simulink model "Distrubted_Settling_IO"  (R2021b)
settings: Solver=ode15s  StartTime=0.0  StopTime=600  FixedStep=0.01  RelTol=1e-5  AbsTol=1e-8
undefined symbols (not defined in the file or in its folder): Split_1_1, Split_2_1
settings Model: Creator=ielulf  LastModifiedBy=javanmcguckin
settings SolverCC: AutoScaleAbsTol=off  AlgebraicLoopSolver=TrustRegion
settings DataIOCC: InitialState=xFinal  SaveFormat=Array  SignalLoggingSaveFormat=ModelDataLogs  SaveOutput=off  ReturnWorkspaceOutputs=off  TimeSaveName=t  SignalLoggingName=sigsOut  OutputTimes=[0:(1/96):609]
settings OptimizationCC: BlockReduction=off  BooleanDataType=off  OptimizeBlockIOStorage=off  BufferReuse=off  GlobalBufferReuse=off  ExpressionFolding=off  ExpressionDepthLimit=2147483647  LocalBlockOutputs=off  InitFltsAndDblsToZero=on  LifeSpan=inf
settings DebuggingCC: SaveWithParameterizedLinksMsg=none  UnderspecifiedInitializationDetection=Classic  MergeDetectMultiDrivingBlocksExec=none  SignalResolutionControl=TryResolveAllWithWarning  InheritedTsInSrcMsg=none  MultiTaskDSMMsg=warning  MultiTaskCondExecSysMsg=none  FcnCallInpInsideContextMsg=warning  UnconnectedOutputMsg=none  StateNameClashWarn=warning  SFUnexpectedBacktrackingDiag=warning  SFNoUnconditionalDefaultTransitionDiag=warning  SFExecutionAtInitializationDiag=none  SFMachineParentedDataDiag=warning  ArithmeticOperatorsInVariantConditions=warning
settings HardwareCC: ProdBitPerPointer=32  ProdBitPerSizeT=32  ProdBitPerPtrDiffT=32  ProdLargestAtomicFloat=None  ProdIntDivRoundTo=Undefined  ProdEndianess=Unspecified  ProdWordSize=32  ProdHWDeviceType=32-bit Generic  TargetUnknown=on
settings ModelReferenceCC: PropagateSignalLabelsOutOfModel=off
settings SFSimCC: SimUseLocalCustomCode=off  CustomCodeUndefinedFunction=UseInterfaceOnly
settings RTWCC: TemplateMakefile=grt_unix.tmf  RTWUseLocalCustomCode=off
settings CodeAppCC: StateflowObjectComments=on
settings GRTTargetCC: TargetFcnLib=ansi_tfl_tmw.mat  TargetLangStandard=C89/C90 (ANSI)  CombineOutputUpdateFcns=off  GRTInterface=on
settings ConfigComp: CovMetricSettings=dw  CovSaveCumulativeToWorkspaceVar=on  CovSaveSingleToWorkspaceVar=on  CovExternalEMLEnable=off

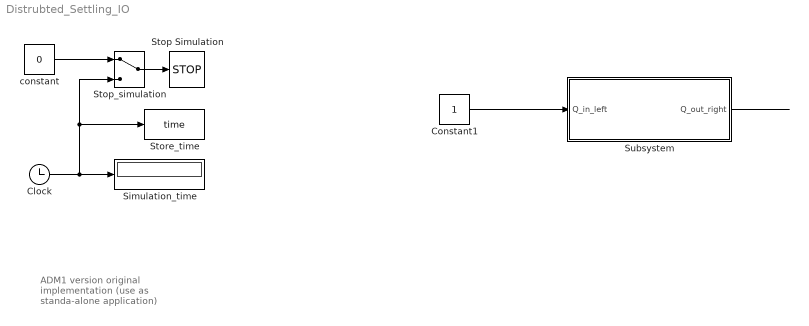
== system Distrubted_Settling_IO ==
  note: ADM1 version
      | original implementation
      | (use as standa-alone application)
  " constant" : Constant  Value=0
  Clock : Clock
  Constant1 : Constant
  Simulation_time : Display
  Stop Simulation : Stop
  Stop_simulation : ManualSwitch
  Store_time : ToWorkspace  VariableName=time
  Subsystem : Subsystem
  wires:
  Clock/1 -> Simulation_time/1, Stop_simulation/2, Store_time/1
  Stop_simulation/1 -> Stop Simulation/1
  " constant"/1 -> Stop_simulation/1
  Constant1/1 -> Subsystem/1(Q_in_left)
  Subsystem/1(Q_out_right) -> ?

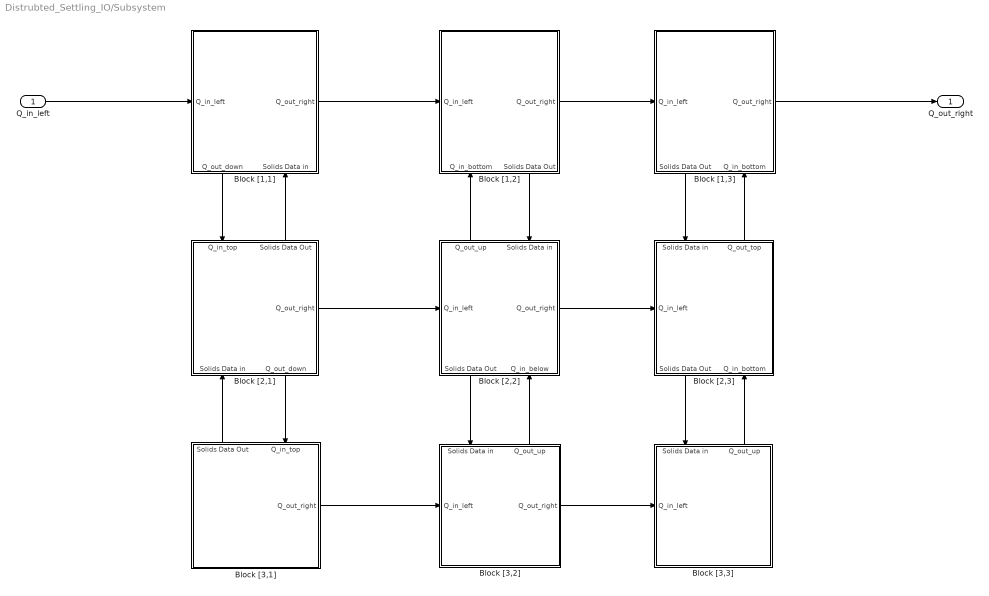
== system Distrubted_Settling_IO/Subsystem ==
  Q_in_left : Inport
  Block [1,1] : Subsystem
      settings: PortSchema="{\"entries\":[{\"content\":{\"sides\":[{\"content\":{\"connectorIds\":[\"In1\"]},\"type\":\"ConnectorPlacement.EquallySpacedRectSide\",\"uuid\":\"2b9ec2c5-2346-4716-8f77-26cfae708b75\"},{\"content\":{\"connectorIds\":[\"Out1\"],\"side\":\"RIGHT\"},\"type\":\"ConnectorPlacement.EquallySpacedRectSide\",\"uuid\":\"6f8825a3-51a4-4a9b-b2dd-ef4b1cf0d0ba\"},{\"content\":{\"connectorIds\":[],\"side\":\"TOP\"},\"type\":\"ConnectorPlacement.EquallySpacedRectSide\",\"uuid\":\"b45032d4-615e-469b-9b78-89fa084c4375\"},{\"content\":{\"connectorIds\":[\"Out2\",\"In2\"],\"side\":\"BOTTOM\"},\"type\":\"ConnectorPlacement.EquallySpacedRectSide\",\"uuid\":\"d5d8c6f1-1ff5-49da-af34-fac996f1665a\"}]},\"type\":\"ConnectorPlacement.EquallySpacedConnector\",\"uuid\":\"ae12b195-59d8-427e-9be1-69bc4b3728a5\"}],\"packageUris\":[\"http://schema.mathworks.com/mf0/Connector/R2020b\"],\"version\":\"1.0\"}"
  Block [1,2] : Subsystem
      settings: PortSchema="{\"entries\":[{\"content\":{\"sides\":[{\"content\":{\"connectorIds\":[\"In1\"]},\"type\":\"ConnectorPlacement.EquallySpacedRectSide\",\"uuid\":\"2b9ec2c5-2346-4716-8f77-26cfae708b75\"},{\"content\":{\"connectorIds\":[\"Out1\"],\"side\":\"RIGHT\"},\"type\":\"ConnectorPlacement.EquallySpacedRectSide\",\"uuid\":\"6f8825a3-51a4-4a9b-b2dd-ef4b1cf0d0ba\"},{\"content\":{\"connectorIds\":[],\"side\":\"TOP\"},\"type\":\"ConnectorPlacement.EquallySpacedRectSide\",\"uuid\":\"b45032d4-615e-469b-9b78-89fa084c4375\"},{\"content\":{\"connectorIds\":[\"In2\",\"Out2\"],\"side\":\"BOTTOM\"},\"type\":\"ConnectorPlacement.EquallySpacedRectSide\",\"uuid\":\"c255c3dc-4fb4-4a4d-908b-3c1bba827588\"}]},\"type\":\"ConnectorPlacement.EquallySpacedConnector\",\"uuid\":\"ae12b195-59d8-427e-9be1-69bc4b3728a5\"}],\"packageUris\":[\"http://schema.mathworks.com/mf0/Connector/R2020b\"],\"version\":\"1.0\"}"
  Block [1,3] : Subsystem
      settings: PortSchema="{\"entries\":[{\"content\":{\"sides\":[{\"content\":{\"connectorIds\":[\"In1\"]},\"type\":\"ConnectorPlacement.EquallySpacedRectSide\",\"uuid\":\"2b9ec2c5-2346-4716-8f77-26cfae708b75\"},{\"content\":{\"connectorIds\":[\"Out1\"],\"side\":\"RIGHT\"},\"type\":\"ConnectorPlacement.EquallySpacedRectSide\",\"uuid\":\"6f8825a3-51a4-4a9b-b2dd-ef4b1cf0d0ba\"},{\"content\":{\"connectorIds\":[],\"side\":\"TOP\"},\"type\":\"ConnectorPlacement.EquallySpacedRectSide\",\"uuid\":\"b45032d4-615e-469b-9b78-89fa084c4375\"},{\"content\":{\"connectorIds\":[\"Out2\",\"In2\"],\"side\":\"BOTTOM\"},\"type\":\"ConnectorPlacement.EquallySpacedRectSide\",\"uuid\":\"c6fd4661-f5fa-4e09-ac4d-c40a325ebb1e\"}]},\"type\":\"ConnectorPlacement.EquallySpacedConnector\",\"uuid\":\"ae12b195-59d8-427e-9be1-69bc4b3728a5\"}],\"packageUris\":[\"http://schema.mathworks.com/mf0/Connector/R2020b\"],\"version\":\"1.0\"}"
  Block [2,1] : Subsystem
      settings: PortSchema="{\"entries\":[{\"content\":{\"sides\":[{\"content\":{\"connectorIds\":[]},\"type\":\"ConnectorPlacement.EquallySpacedRectSide\",\"uuid\":\"3629ef0d-6d1b-4007-aa46-2d78e3d7de39\"},{\"content\":{\"connectorIds\":[\"Out1\"],\"side\":\"RIGHT\"},\"type\":\"ConnectorPlacement.EquallySpacedRectSide\",\"uuid\":\"902c1b28-6e40-40dc-9ba4-02f520de612f\"},{\"content\":{\"connectorIds\":[\"In1\",\"Out3\"],\"side\":\"TOP\"},\"type\":\"ConnectorPlacement.EquallySpacedRectSide\",\"uuid\":\"32048d77-21e8-4d7f-b37a-aa0fba1296d3\"},{\"content\":{\"connectorIds\":[\"In2\",\"Out2\"],\"side\":\"BOTTOM\"},\"type\":\"ConnectorPlacement.EquallySpacedRectSide\",\"uuid\":\"7ea0cf0e-949f-46a7-b1ef-2c29e41bdeea\"}]},\"type\":\"ConnectorPlacement.EquallySpacedConnector\",\"uuid\":\"783f8f0c-f046-4b3b-a07c-ac2bcfa72a90\"}],\"packageUris\":[\"http://schema.mathworks.com/mf0/Connector/R2020b\"],\"version\":\"1.0\"}"
  Block [2,2] : Subsystem
      settings: PortSchema="{\"entries\":[{\"content\":{\"sides\":[{\"content\":{\"connectorIds\":[\"In1\"]},\"type\":\"ConnectorPlacement.EquallySpacedRectSide\",\"uuid\":\"49108942-846e-4f10-a565-9a363346b2ee\"},{\"content\":{\"connectorIds\":[\"Out1\"],\"side\":\"RIGHT\"},\"type\":\"ConnectorPlacement.EquallySpacedRectSide\",\"uuid\":\"12efabec-6f68-4acd-88b6-a333148dee6c\"},{\"content\":{\"connectorIds\":[\"Out3\",\"In2\"],\"side\":\"TOP\"},\"type\":\"ConnectorPlacement.EquallySpacedRectSide\",\"uuid\":\"4d5dbabd-8754-411c-8b88-a1dca35fc46d\"},{\"content\":{\"connectorIds\":[\"Out2\",\"In3\"],\"side\":\"BOTTOM\"},\"type\":\"ConnectorPlacement.EquallySpacedRectSide\",\"uuid\":\"6311604b-5e77-49d3-b6da-7ee01c36d0f1\"}]},\"type\":\"ConnectorPlacement.EquallySpacedConnector\",\"uuid\":\"2bdac1b1-172b-46d0-a20b-b916e0c0b218\"}],\"packageUris\":[\"http://schema.mathworks.com/mf0/Connector/R2020b\"],\"version\":\"1.0\"}"
  Block [2,3] : Subsystem
      settings: PortSchema="{\"entries\":[{\"content\":{\"sides\":[{\"content\":{\"connectorIds\":[\"In1\"]},\"type\":\"ConnectorPlacement.EquallySpacedRectSide\",\"uuid\":\"482fbcbb-9155-4fc8-9601-0ed92cde34b4\"},{\"content\":{\"connectorIds\":[],\"side\":\"RIGHT\"},\"type\":\"ConnectorPlacement.EquallySpacedRectSide\",\"uuid\":\"966a36b1-158b-4266-8167-7a28a80d741e\"},{\"content\":{\"connectorIds\":[\"In2\",\"Out2\"],\"side\":\"TOP\"},\"type\":\"ConnectorPlacement.EquallySpacedRectSide\",\"uuid\":\"4202d0b1-6626-47db-a2e1-ad8e088ff7d9\"},{\"content\":{\"connectorIds\":[\"Out1\",\"In3\"],\"side\":\"BOTTOM\"},\"type\":\"ConnectorPlacement.EquallySpacedRectSide\",\"uuid\":\"461d971e-62b1-46e7-bd8e-21338c52363b\"}]},\"type\":\"ConnectorPlacement.EquallySpacedConnector\",\"uuid\":\"aeaa18e4-b5a1-4196-839a-a6726a008bcb\"}],\"packageUris\":[\"http://schema.mathworks.com/mf0/Connector/R2020b\"],\"version\":\"1.0\"}"
  Block [3,1] : Subsystem
      settings: PortSchema="{\"entries\":[{\"content\":{\"sides\":[{\"content\":{\"connectorIds\":[]},\"type\":\"ConnectorPlacement.EquallySpacedRectSide\",\"uuid\":\"dae4b3ee-e133-472e-b2ea-e36730571ee8\"},{\"content\":{\"connectorIds\":[\"Out1\"],\"side\":\"RIGHT\"},\"type\":\"ConnectorPlacement.EquallySpacedRectSide\",\"uuid\":\"e23d6f38-e3a9-4ba0-b1b2-a35021c5cf93\"},{\"content\":{\"connectorIds\":[\"Out2\",\"In1\"],\"side\":\"TOP\"},\"type\":\"ConnectorPlacement.EquallySpacedRectSide\",\"uuid\":\"a0192f9c-1394-43a9-92b6-f99a3e548f6c\"}]},\"type\":\"ConnectorPlacement.EquallySpacedConnector\",\"uuid\":\"83d38208-dd44-485f-8397-f334694b3944\"}],\"packageUris\":[\"http://schema.mathworks.com/mf0/Connector/R2020b\"],\"version\":\"1.0\"}"
  Block [3,2] : Subsystem
      settings: PortSchema="{\"entries\":[{\"content\":{\"sides\":[{\"content\":{\"connectorIds\":[\"In1\"]},\"type\":\"ConnectorPlacement.EquallySpacedRectSide\",\"uuid\":\"2b9ec2c5-2346-4716-8f77-26cfae708b75\"},{\"content\":{\"connectorIds\":[\"Out1\"],\"side\":\"RIGHT\"},\"type\":\"ConnectorPlacement.EquallySpacedRectSide\",\"uuid\":\"6f8825a3-51a4-4a9b-b2dd-ef4b1cf0d0ba\"},{\"content\":{\"connectorIds\":[\"In2\",\"Out2\"],\"side\":\"TOP\"},\"type\":\"ConnectorPlacement.EquallySpacedRectSide\",\"uuid\":\"b45032d4-615e-469b-9b78-89fa084c4375\"}]},\"type\":\"ConnectorPlacement.EquallySpacedConnector\",\"uuid\":\"ae12b195-59d8-427e-9be1-69bc4b3728a5\"}],\"packageUris\":[\"http://schema.mathworks.com/mf0/Connector/R2020b\"],\"version\":\"1.0\"}"
  Block [3,3] : Subsystem
      settings: PortSchema="{\"entries\":[{\"content\":{\"sides\":[{\"content\":{\"connectorIds\":[\"In1\"]},\"type\":\"ConnectorPlacement.EquallySpacedRectSide\",\"uuid\":\"2945329d-4d23-477b-9be7-b4c63a0bfb0a\"},{\"content\":{\"connectorIds\":[],\"side\":\"RIGHT\"},\"type\":\"ConnectorPlacement.EquallySpacedRectSide\",\"uuid\":\"7476eda5-2d2c-4a8f-8f7c-d1792aee789c\"},{\"content\":{\"connectorIds\":[\"In2\",\"Out1\"],\"side\":\"TOP\"},\"type\":\"ConnectorPlacement.EquallySpacedRectSide\",\"uuid\":\"7de1c60b-266e-4668-808d-5560ef68021a\"}]},\"type\":\"ConnectorPlacement.EquallySpacedConnector\",\"uuid\":\"0844fd89-a54f-4951-a866-f1bf8a22511d\"}],\"packageUris\":[\"http://schema.mathworks.com/mf0/Connector/R2020b\"],\"version\":\"1.0\"}"
  Q_out_right : Outport
  wires:
  Block [1,3]/2(Solids Data Out) -> Block [2,3]/2(Solids Data in)
  Block [3,3]/1(Q_out_up) -> Block [2,3]/3(Q_in_bottom)
  Block [2,3]/1(Solids Data Out) -> Block [3,3]/2(Solids Data in)
  Block [1,1]/1(Q_out_right) -> Block [1,2]/1(Q_in_left)
  Block [1,2]/2(Solids Data Out) -> Block [2,2]/2(Solids Data in)
  Block [3,1]/2(Solids Data Out) -> Block [2,1]/2(Solids Data in)
  Block [2,2]/1(Q_out_right) -> Block [2,3]/1(Q_in_left)
  Block [2,2]/2(Solids Data Out) -> Block [3,2]/2(Solids Data in)
  Block [2,2]/3(Q_out_up) -> Block [1,2]/2(Q_in_bottom)
  Block [3,2]/2(Q_out_up) -> Block [2,2]/3(Q_in_below)
  Block [2,1]/1(Q_out_right) -> Block [2,2]/1(Q_in_left)
  Block [1,1]/2(Q_out_down) -> Block [2,1]/1(Q_in_top)
  Q_in_left/1 -> Block [1,1]/1(Q_in_left)
  Block [3,2]/1(Q_out_right) -> Block [3,3]/1(Q_in_left)
  Block [2,1]/3(Solids Data Out) -> Block [1,1]/2(Solids Data in)
  Block [1,3]/1(Q_out_right) -> Q_out_right/1
  Block [3,1]/1(Q_out_right) -> Block [3,2]/1(Q_in_left)
  Block [2,3]/2(Q_out_top) -> Block [1,3]/2(Q_in_bottom)
  Block [2,1]/2(Q_out_down) -> Block [3,1]/1(Q_in_top)
  Block [1,2]/1(Q_out_right) -> Block [1,3]/1(Q_in_left)

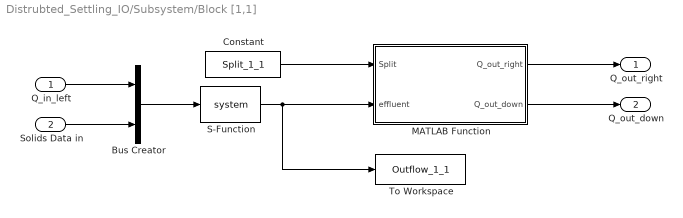
== system Distrubted_Settling_IO/Subsystem/Block [1,1] ==
  Q_in_left : Inport
  Solids Data in : Inport  Port=2
  Bus Creator : BusCreator  Inputs=2
  Constant : Constant  Value=Split_1_1
  MATLAB Function : MATLAB Function  TreatAsAtomicUnit=on
  S-Function : S-Function  SFunctionDeploymentMode=off  EnableBusSupport=off
  To Workspace : ToWorkspace  VariableName=Outflow_1_1  SaveFormat=Timeseries  SampleTime=-1
  Q_out_right : Outport
  Q_out_down : Outport  Port=2
  wires:
  Q_in_left/1 -> Bus Creator/1
  Solids Data in/1 -> Bus Creator/2
  Bus Creator/1 -> S-Function/1
  S-Function/1 -> MATLAB Function/2(effluent), To Workspace/1
  MATLAB Function/1(Q_out_right) -> Q_out_right/1
  Constant/1 -> MATLAB Function/1(Split)
  MATLAB Function/2(Q_out_down) -> Q_out_down/1

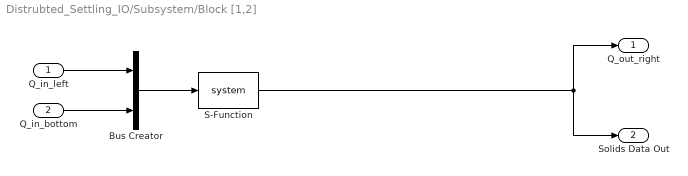
== system Distrubted_Settling_IO/Subsystem/Block [1,2] ==
  Q_in_left : Inport
  Q_in_bottom : Inport  Port=2
  Bus Creator : BusCreator  Inputs=2
  S-Function : S-Function  SFunctionDeploymentMode=off  EnableBusSupport=off
  Q_out_right : Outport
  Solids Data Out : Outport  Port=2
  wires:
  Q_in_left/1 -> Bus Creator/1
  Bus Creator/1 -> S-Function/1
  S-Function/1 -> Solids Data Out/1, Q_out_right/1
  Q_in_bottom/1 -> Bus Creator/2

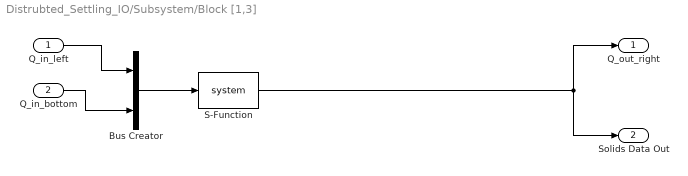
== system Distrubted_Settling_IO/Subsystem/Block [1,3] ==
  Q_in_left : Inport
  Q_in_bottom : Inport  Port=2
  Bus Creator : BusCreator  Inputs=2
  S-Function : S-Function  SFunctionDeploymentMode=off  EnableBusSupport=off
  Q_out_right : Outport
  Solids Data Out : Outport  Port=2
  wires:
  Q_in_left/1 -> Bus Creator/1
  Bus Creator/1 -> S-Function/1
  S-Function/1 -> Solids Data Out/1, Q_out_right/1
  Q_in_bottom/1 -> Bus Creator/2

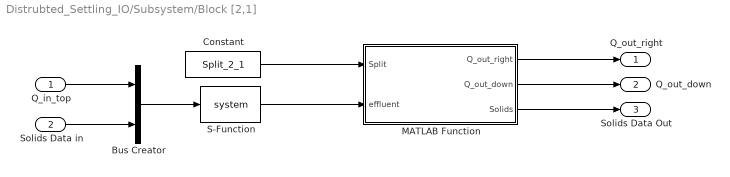
== system Distrubted_Settling_IO/Subsystem/Block [2,1] ==
  Q_in_top : Inport
  Solids Data in : Inport  Port=2
  Bus Creator : BusCreator  Inputs=2
  Constant : Constant  Value=Split_2_1
  MATLAB Function : MATLAB Function  TreatAsAtomicUnit=on
  S-Function : S-Function  SFunctionDeploymentMode=off  EnableBusSupport=off
  Q_out_right : Outport
  Q_out_down : Outport  Port=2
  Solids Data Out : Outport  Port=3
  wires:
  Q_in_top/1 -> Bus Creator/1
  Solids Data in/1 -> Bus Creator/2
  Bus Creator/1 -> S-Function/1
  S-Function/1 -> MATLAB Function/2(effluent)
  Constant/1 -> MATLAB Function/1(Split)
  MATLAB Function/2(Q_out_down) -> Q_out_down/1
  MATLAB Function/1(Q_out_right) -> Q_out_right/1
  MATLAB Function/3(Solids) -> Solids Data Out/1

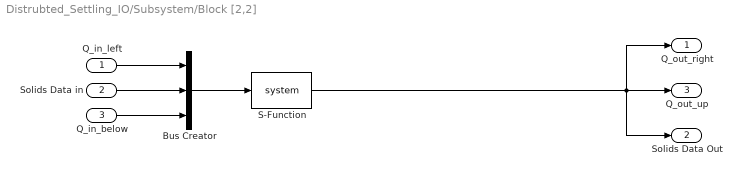
== system Distrubted_Settling_IO/Subsystem/Block [2,2] ==
  Q_in_left : Inport
  Solids Data in : Inport  Port=2
  Q_in_below : Inport  Port=3
  Bus Creator : BusCreator  Inputs=3
  S-Function : S-Function  SFunctionDeploymentMode=off  EnableBusSupport=off
  Q_out_right : Outport
  Solids Data Out : Outport  Port=2
  Q_out_up : Outport  Port=3
  wires:
  Q_in_left/1 -> Bus Creator/1
  Solids Data in/1 -> Bus Creator/2
  Bus Creator/1 -> S-Function/1
  S-Function/1 -> Q_out_up/1, Solids Data Out/1, Q_out_right/1
  Q_in_below/1 -> Bus Creator/3

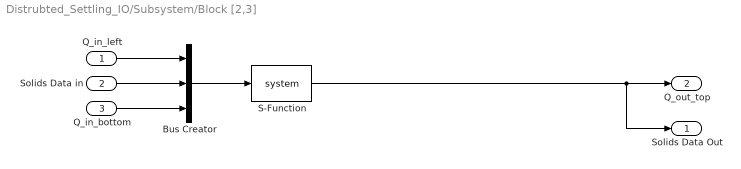
== system Distrubted_Settling_IO/Subsystem/Block [2,3] ==
  Q_in_left : Inport
  Solids Data in : Inport  Port=2
  Q_in_bottom : Inport  Port=3
  Bus Creator : BusCreator  Inputs=3
  S-Function : S-Function  SFunctionDeploymentMode=off  EnableBusSupport=off
  Solids Data Out : Outport
  Q_out_top : Outport  Port=2
  wires:
  Q_in_left/1 -> Bus Creator/1
  Solids Data in/1 -> Bus Creator/2
  Bus Creator/1 -> S-Function/1
  S-Function/1 -> Q_out_top/1, Solids Data Out/1
  Q_in_bottom/1 -> Bus Creator/3

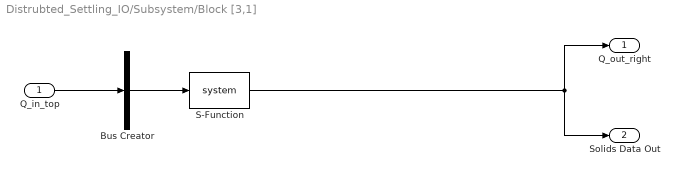
== system Distrubted_Settling_IO/Subsystem/Block [3,1] ==
  Q_in_top : Inport
  Bus Creator : BusCreator  Inputs=1
  S-Function : S-Function  SFunctionDeploymentMode=off  EnableBusSupport=off
  Q_out_right : Outport
  Solids Data Out : Outport  Port=2
  wires:
  Q_in_top/1 -> Bus Creator/1
  Bus Creator/1 -> S-Function/1
  S-Function/1 -> Solids Data Out/1, Q_out_right/1

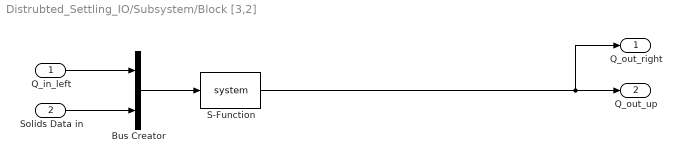
== system Distrubted_Settling_IO/Subsystem/Block [3,2] ==
  Q_in_left : Inport
  Solids Data in : Inport  Port=2
  Bus Creator : BusCreator  Inputs=2
  S-Function : S-Function  SFunctionDeploymentMode=off  EnableBusSupport=off
  Q_out_right : Outport
  Q_out_up : Outport  Port=2
  wires:
  Q_in_left/1 -> Bus Creator/1
  Solids Data in/1 -> Bus Creator/2
  Bus Creator/1 -> S-Function/1
  S-Function/1 -> Q_out_up/1, Q_out_right/1

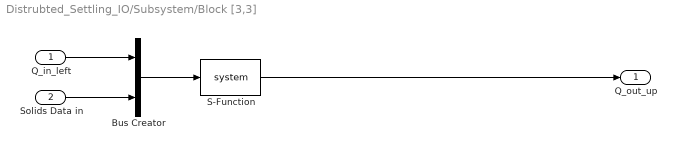
== system Distrubted_Settling_IO/Subsystem/Block [3,3] ==
  Q_in_left : Inport
  Solids Data in : Inport  Port=2
  Bus Creator : BusCreator  Inputs=2
  S-Function : S-Function  SFunctionDeploymentMode=off  EnableBusSupport=off
  Q_out_up : Outport
  wires:
  Q_in_left/1 -> Bus Creator/1
  Solids Data in/1 -> Bus Creator/2
  Bus Creator/1 -> S-Function/1
  S-Function/1 -> Q_out_up/1

== matlab function Distrubted_Settling_IO/Subsystem/Block [2,1]/MATLAB Function ==
  data: Split input; effluent input; Q_out_right output; Q_out_down output; Solids output
function [Q_out_right,Q_out_down,Solids] = fcn(Split, effluent)


%% Correcting Effluent for SRT
effluent(:,13:24) = (effluent(:,13:24))*V_liq./(effluent(:,25)*T_res);
effluent(:,33)    = (effluent(:,33))*V_liq./(effluent(:,25)*T_res);

%% Set up blank matrix to fill with values from block [1,1] effluent
Storage_flow               = zeros(length(effluent),94);

% S_Su, S_aa, S_fa, S_va, S_bu, S_pro, S_ac, S_h2, S_ch4, S_IC, S_IN, S_I,
% X_c, X_ch, X_pr, X_li, X_su, X_aa, X_fa, X_c4, X_pro, X_ac, X_h2, X_I,
% Q_in, T
Storage_flow(:,[1:26]) = effluent(:,[1:26]);

% MS (Mineral Solids)
Storage_flow(:,[27]) = effluent(:,[33]);

% Na, K, Cl
Storage_flow(:,[46:48])=effluent(:,[75:77]);

% Splitting the flow rate between the two streams flowing out
Storage_flow_right = Storage_flow;
Storage_flow_right(:,[25]) = Storage_flow_right(:,[25]).* Split;

Storage_flow_down = Storage_flow;
Storage_flow_down(:,[25]) = Storage_flow_right(:,[25]).*(1- Split);


%% SOLIDS DATA

Storage_Solids = zeros(length(effluent),20);

% X_c, X_ch, X_pr, X_li, X_su, X_aa, X_fa, X_c4, X_pro, X_ac, X_h2, X_I
Storage_Solids(:,[1:12]) = effluent(:,([13:24]);
% MS
Storage_Solids(:,[13]) = effluent(:,([33]);

VSS_out = sum(effluent(:,14:16),2)/1.5686 + ...
          sum(effluent(:,17:23),2)/1.3072 + ...
          effluent(:,24)/1.5686;

TSS_out = effluent[:,33] + VSS_out;


%% Outputs

Q_out_right     = Storage_flow_right;
Q_out_down      = Storage_flow_down;
Solids          = Storage_Solids;

== matlab function Distrubted_Settling_IO/Subsystem/Block [1,1]/MATLAB Function ==
  data: Split input; effluent input; Q_out_right output; Q_out_down output
function [Q_out_right,Q_out_down] = fcn(Split, effluent)


%% FLOWS
% Set up blank matrix to fill with values from block [1,1] effluent
Storage_flow               = zeros(length(effluent),94);

% S_Su, S_aa, S_fa, S_va, S_bu, S_pro, S_ac, S_h2, S_ch4, S_IC, S_IN, S_I,
% X_c, X_ch, X_pr, X_li, X_su, X_aa, X_fa, X_c4, X_pro, X_ac, X_h2, X_I,
% Q_in, T
Storage_flow(:,[1:26]) = effluent(:,[1:26]);

% MS (Mineral Solids)
Storage_flow(:,[27]) = effluent(:,[33]);

% Na, K, Cl
Storage_flow(:,[46:48])=effluent(:,[75:77]);

Storage_flow_right = Storage_flow;
Storage_flow_right(:,[25]) = Storage_flow_right(:,[25]).* Split;

Storage_flow_down = Storage_flow;
Storage_flow_down(:,[25]) = Storage_flow_right(:,[25]).*(1- Split);


%% SOLIDS DATA
% Not applicable for this block.

%% Outputs

Q_out_right = Storage_flow_right;
Q_out_down = Storage_flow_down;
